simulink model "test_supervisorV2"  (R2023b)
settings: Solver=FixedStepDiscrete  StartTime=0.0  StopTime=inf  FixedStep=1e-3  RelTol=1e-3  EnableMultiTasking=on
undefined symbols (not defined in the file): ControlModes, MotionControlInitConf, SupervisorEvents
libraries: simulink x1
settings Model: DataDictionary=common.sldd  Creator=mfussi  LastModifiedBy=mfussi
settings SolverCC: ConcurrentTasks=on  AutoInsertRateTranBlk=on  InsertRTBMode=Never (minimum delay)
settings DataIOCC: SaveOutput=off  SignalLogging=off  DSMLogging=off  StreamToWks=off  SaveTime=off  ReturnWorkspaceOutputs=off
settings OptimizationCC: DefaultParameterBehavior=Inlined  UseDivisionForNetSlopeComputation=on  GainParamInheritBuiltInType=on  UseFloatMulNetSlope=on  InlineInvariantSignals=on  EnhancedBackFolding=on  NoFixptDivByZeroProtection=on  EfficientFloat2IntCast=on  OptimizeBlockOrder=speed  DifferentSizesBufferReuse=on  OptimizationCustomize=off  EfficientTunableParamExpr=on
settings DebuggingCC: ParameterTunabilityLossMsg=error
settings HardwareCC: ProdBitPerPointer=32  ProdBitPerSizeT=32  ProdBitPerPtrDiffT=32  ProdLargestAtomicInteger=Long  ProdLargestAtomicFloat=Double  ProdWordSize=32  ProdLongLongMode=on  ProdHWDeviceType=ARM Compatible->ARM Cortex-M
settings SFSimCC: MATLABDynamicMemAlloc=off
settings SFSimCC: SimCustomHeaderCode=|
  | #include "rtw_enable_disable_motors.h"
  | #include "rtw_motor_config.h"
settings SFSimCC: SimUserSources=|
  | rtw_enable_disable_motors.c
  | rtw_motor_config.c
settings RTWCC: Description=Embedded Coder  SystemTargetFile=ert.tlc  GenCodeOnly=on  TemplateMakefile=ert_default_tmf  RTWUseSimCustomCode=on
settings RTWCC: CustomHeaderCode=|
  | #include "rtw_enable_disable_motors.h"
  | #include "rtw_motor_config.h"
settings RTWCC: CustomSource=|
  | rtw_enable_disable_motors.c
  | rtw_motor_config.c
settings CodeAppCC: ForceParamTrailComments=on  IgnoreCustomStorageClasses=off  OperatorAnnotations=on  SimulinkDataObjDesc=on  SFDataObjDesc=on  InsertBlockDesc=on
settings ERTTargetCC: TargetLangStandard=C99 (ISO)  CodeReplacementLibrary=ARM Cortex-M,iCubTech  GenerateSampleERTMain=on  SuppressErrorStatus=on  CodeInterfacePackaging=Reusable function  SupportNonFinite=off  InlinedParameterPlacement=NonHierarchical  RootIOFormat=Structure reference  ERTCustomFileTemplate=example_file_process.tlc

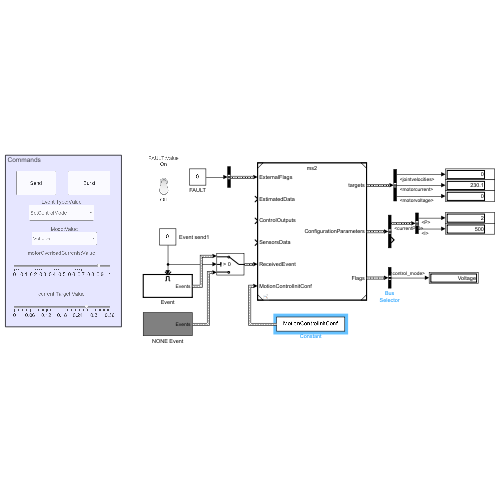
[thumbnail: Simulink's stored preview of the top-level diagram]
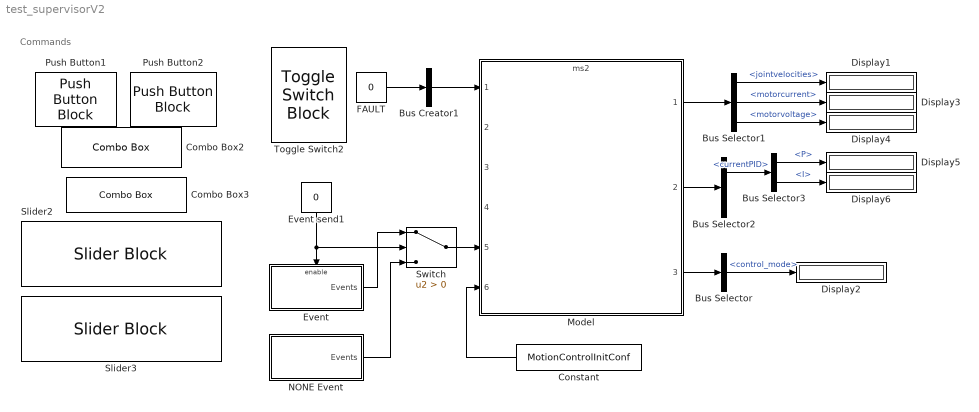
== system test_supervisorV2 ==
  note: Commands
  Bus Creator1 : BusCreator  Inputs=1  OutDataTypeStr=Bus: ExternalFlags  NonVirtualBus=on
      settings: InheritFromInputs=off
  Bus Selector : BusSelector  OutputSignals=control_mode
  Bus Selector1 : BusSelector  OutputSignals=jointvelocities,motorcurrent,motorvoltage
  Bus Selector2 : BusSelector  OutputSignals=pids.currentPID,thresholds
  Bus Selector3 : BusSelector  OutputSignals=P,I
  Combo Box2 : ComboBox  SelectedLabel=SetControlMode  UseEnumeratedDataType=on  EnumeratedDataType=SupervisorEvents
      settings: Values={{'None', 'SetLimit', 'SetControlMode', 'SetMotorConfig', 'SetPid', 'SetTarget'}, [0 1 2 5 3 4]}
  Combo Box3 : ComboBox  SelectedLabel=Voltage  UseEnumeratedDataType=on  EnumeratedDataType=ControlModes
      settings: Values={{'NotConfigured', 'Idle', 'Position', 'PositionDirect', 'Current', 'Velocity', 'Voltage', 'Torque', 'HwFaultCM'}, [0 1 2 3 4 5 6 7 8]}
  Constant : Constant  Value=MotionControlInitConf  OutDataTypeStr=Bus: ActuatorConfiguration
  Display{1..6} (6 alike) : Display
  Event : Subsystem
  Event send1 : Constant  Value=0
  FAULT : Constant  Value=0  OutDataTypeStr=Inherit: Inherit via back propagation
  Model : ModelReference  ModelNameDialog=ms2.slx  SimulationMode=Normal  ModelReferenceVersion=1.148
  NONE Event : Subsystem
  Push Button1 : PushButtonBlock  ButtonText=Send  OffValue=0.000000
  Push Button2 : PushButtonBlock  ButtonText=Burst  ButtonType=Latch  OffValue=0.000000
  Slider2 : SliderBlock  ScaleMax=1
  Slider3 : SliderBlock  ScaleMax=0.36
  Switch : Switch  Criteria=u2 > Threshold  SaturateOnIntegerOverflow=off  InputSameDT=off
  Toggle Switch2 : ToggleSwitchBlock
      settings: Values={{'Off', 'On'}, [0 1]}
  wires:
  Event/1(Events) -> Switch/1
  FAULT/1 -> Bus Creator1/1
  Bus Creator1/1 -> Model/1
  Model/3 -> Bus Selector/1
  Bus Selector/1 -> Display2/1  "<control_mode>"
  Switch/1 -> Model/5
  Event send1/1 -> Switch/2, Event/Enable
  NONE Event/1(Events) -> Switch/3
  Model/1 -> Bus Selector1/1
  Bus Selector1/1 -> Display1/1  "<jointvelocities>"
  Bus Selector1/2 -> Display3/1  "<motorcurrent>"
  Bus Selector1/3 -> Display4/1  "<motorvoltage>"
  Bus Selector2/1 -> Bus Selector3/1  "<currentPID>"
  Constant/1 -> Model/6
  Model/2 -> Bus Selector2/1
  Bus Selector3/1 -> Display5/1  "<P>"
  Bus Selector3/2 -> Display6/1  "<I>"

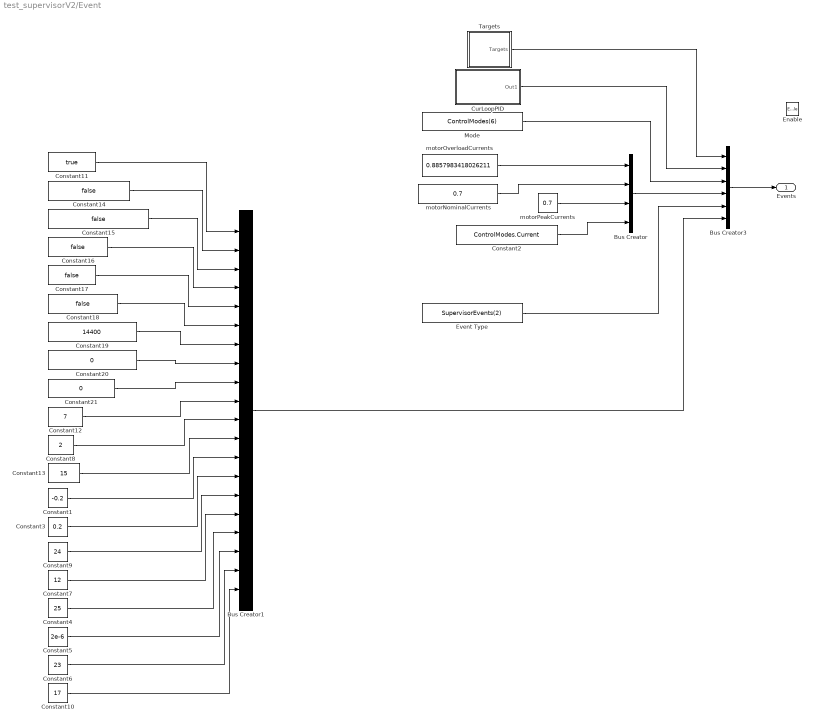
== system test_supervisorV2/Event ==
  Enable : EnablePort
  Bus Creator : BusCreator  Inputs=4  OutDataTypeStr=Bus: SupervisorInputLimits
  Bus Creator1 : BusCreator  Inputs=20  OutDataTypeStr=Bus: MotorConfiguration  NonVirtualBus=on
      settings: InheritFromInputs=off
  Bus Creator3 : BusCreator  Inputs=6  OutDataTypeStr=Bus: SupervisorReceivedEvents  NonVirtualBus=on
      settings: InheritFromInputs=off
  Constant1 : Constant  Value=-0.2  OutDataTypeStr=single
  Constant10 : Constant  Value=17  OutDataTypeStr=single
  Constant11 : Constant  Value=true  OutDataTypeStr=boolean
  Constant12 : Constant  Value=7  OutDataTypeStr=uint8
  Constant13 : Constant  Value=15  OutDataTypeStr=single
  Constant{14..18} (5 alike) : Constant  Value=false  OutDataTypeStr=boolean
  Constant19 : Constant  Value=14400  OutDataTypeStr=int16
  Constant2 : Constant  Value=ControlModes.Current  OutDataTypeStr=Enum: ControlModes
  Constant20 : Constant  Value=0  OutDataTypeStr=int16
  Constant21 : Constant  Value=0  OutDataTypeStr=uint8
  Constant3 : Constant  Value=0.2  OutDataTypeStr=single
  Constant4 : Constant  Value=25  OutDataTypeStr=single
  Constant5 : Constant  Value=2e-6  OutDataTypeStr=single
  Constant6 : Constant  Value=23  OutDataTypeStr=single
  Constant7 : Constant  Value=12  OutDataTypeStr=single
  Constant8 : Constant  Value=2  OutDataTypeStr=single
  Constant9 : Constant  Value=24  OutDataTypeStr=single
  CurLoopPID : Subsystem  mask{OutMax=0, OutMin=0, P=2, I=500, D=0, N=10, I0=0, D0=0, shift_factor=0}
      mask prompts: shift_factor "Shift Factor"
  Event Type : Constant  Value=SupervisorEvents(2)  OutDataTypeStr=Enum: SupervisorEvents
  Mode : Constant  Value=ControlModes(6)  OutDataTypeStr=Enum: ControlModes
  Targets : Subsystem
  motorNominalCurrents : Constant  Value=0.7  OutDataTypeStr=single
  motorOverloadCurrents : Constant  Value=0.8857983418026211  OutDataTypeStr=single
  motorPeakCurrents : Constant  Value=0.7  OutDataTypeStr=single
  Events : Outport  OutDataTypeStr=Bus: SupervisorReceivedEvents
  wires:
  Bus Creator/1 -> Bus Creator3/4
  Bus Creator1/1 -> Bus Creator3/6
  Mode/1 -> Bus Creator3/3
  Targets/1(Targets) -> Bus Creator3/1
  Event Type/1 -> Bus Creator3/5
  CurLoopPID/1(Out1) -> Bus Creator3/2
  motorPeakCurrents/1 -> Bus Creator/3
  Constant2/1 -> Bus Creator/4
  motorOverloadCurrents/1 -> Bus Creator/1
  motorNominalCurrents/1 -> Bus Creator/2
  Bus Creator3/1 -> Events/1
  Constant4/1 -> Bus Creator1/17
  Constant6/1 -> Bus Creator1/19
  Constant17/1 -> Bus Creator1/5
  Constant14/1 -> Bus Creator1/2
  Constant8/1 -> Bus Creator1/11
  Constant10/1 -> Bus Creator1/20
  Constant5/1 -> Bus Creator1/18
  Constant11/1 -> Bus Creator1/1
  Constant1/1 -> Bus Creator1/13
  Constant7/1 -> Bus Creator1/16
  Constant9/1 -> Bus Creator1/15
  Constant3/1 -> Bus Creator1/14
  Constant16/1 -> Bus Creator1/4
  Constant13/1 -> Bus Creator1/12
  Constant18/1 -> Bus Creator1/6
  Constant21/1 -> Bus Creator1/9
  Constant12/1 -> Bus Creator1/10
  Constant19/1 -> Bus Creator1/7
  Constant20/1 -> Bus Creator1/8
  Constant15/1 -> Bus Creator1/3

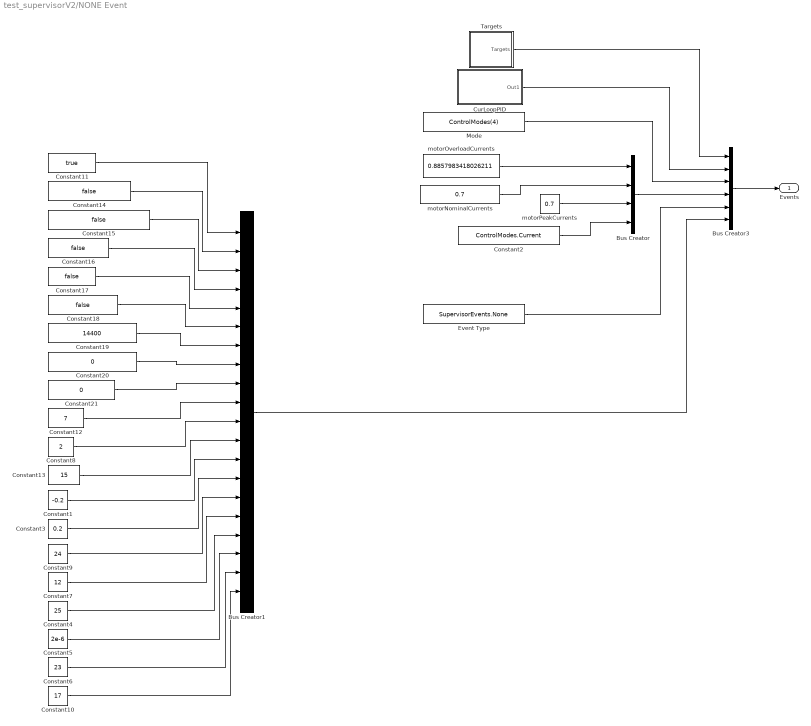
== system test_supervisorV2/NONE Event ==
  Bus Creator : BusCreator  Inputs=4  OutDataTypeStr=Bus: SupervisorInputLimits
  Bus Creator1 : BusCreator  Inputs=20  OutDataTypeStr=Bus: MotorConfiguration  NonVirtualBus=on
      settings: InheritFromInputs=off
  Bus Creator3 : BusCreator  Inputs=6  OutDataTypeStr=Bus: SupervisorReceivedEvents  NonVirtualBus=on
      settings: InheritFromInputs=off
  Constant1 : Constant  Value=-0.2  OutDataTypeStr=single
  Constant10 : Constant  Value=17  OutDataTypeStr=single
  Constant11 : Constant  Value=true  OutDataTypeStr=boolean
  Constant12 : Constant  Value=7  OutDataTypeStr=uint8
  Constant13 : Constant  Value=15  OutDataTypeStr=single
  Constant{14..18} (5 alike) : Constant  Value=false  OutDataTypeStr=boolean
  Constant19 : Constant  Value=14400  OutDataTypeStr=int16
  Constant2 : Constant  Value=ControlModes.Current  OutDataTypeStr=Enum: ControlModes
  Constant20 : Constant  Value=0  OutDataTypeStr=int16
  Constant21 : Constant  Value=0  OutDataTypeStr=uint8
  Constant3 : Constant  Value=0.2  OutDataTypeStr=single
  Constant4 : Constant  Value=25  OutDataTypeStr=single
  Constant5 : Constant  Value=2e-6  OutDataTypeStr=single
  Constant6 : Constant  Value=23  OutDataTypeStr=single
  Constant7 : Constant  Value=12  OutDataTypeStr=single
  Constant8 : Constant  Value=2  OutDataTypeStr=single
  Constant9 : Constant  Value=24  OutDataTypeStr=single
  CurLoopPID : Subsystem  mask{OutMax=0, OutMin=0, P=2, I=500, D=0, N=10, I0=0, D0=0, shift_factor=0}
      mask prompts: shift_factor "Shift Factor"
  Event Type : Constant  Value=SupervisorEvents.None  OutDataTypeStr=Enum: SupervisorEvents
  Mode : Constant  Value=ControlModes(4)  OutDataTypeStr=Enum: ControlModes
  Targets : Subsystem
  motorNominalCurrents : Constant  Value=0.7  OutDataTypeStr=single
  motorOverloadCurrents : Constant  Value=0.8857983418026211  OutDataTypeStr=single
  motorPeakCurrents : Constant  Value=0.7  OutDataTypeStr=single
  Events : Outport  OutDataTypeStr=Bus: SupervisorReceivedEvents
  wires:
  Bus Creator/1 -> Bus Creator3/4
  Bus Creator1/1 -> Bus Creator3/6
  Mode/1 -> Bus Creator3/3
  Targets/1(Targets) -> Bus Creator3/1
  Event Type/1 -> Bus Creator3/5
  CurLoopPID/1(Out1) -> Bus Creator3/2
  motorPeakCurrents/1 -> Bus Creator/3
  Constant2/1 -> Bus Creator/4
  motorOverloadCurrents/1 -> Bus Creator/1
  motorNominalCurrents/1 -> Bus Creator/2
  Bus Creator3/1 -> Events/1
  Constant4/1 -> Bus Creator1/17
  Constant6/1 -> Bus Creator1/19
  Constant17/1 -> Bus Creator1/5
  Constant14/1 -> Bus Creator1/2
  Constant8/1 -> Bus Creator1/11
  Constant10/1 -> Bus Creator1/20
  Constant5/1 -> Bus Creator1/18
  Constant11/1 -> Bus Creator1/1
  Constant1/1 -> Bus Creator1/13
  Constant7/1 -> Bus Creator1/16
  Constant9/1 -> Bus Creator1/15
  Constant3/1 -> Bus Creator1/14
  Constant16/1 -> Bus Creator1/4
  Constant13/1 -> Bus Creator1/12
  Constant18/1 -> Bus Creator1/6
  Constant21/1 -> Bus Creator1/9
  Constant12/1 -> Bus Creator1/10
  Constant19/1 -> Bus Creator1/7
  Constant20/1 -> Bus Creator1/8
  Constant15/1 -> Bus Creator1/3

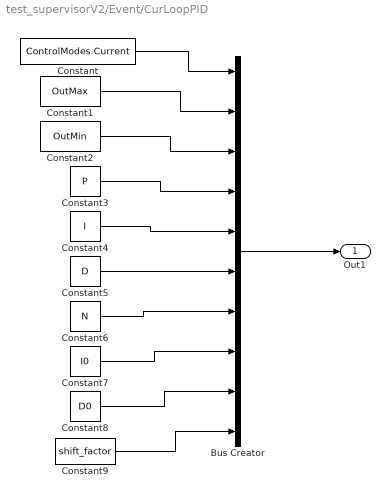
== system test_supervisorV2/Event/CurLoopPID ==
  Bus Creator : BusCreator  Inputs=10  OutDataTypeStr=Bus: PID  NonVirtualBus=on
      settings: InheritFromInputs=off
  Constant : Constant  Value=ControlModes.Current
  Constant1 : Constant  Value=OutMax  OutDataTypeStr=single
  Constant2 : Constant  Value=OutMin  OutDataTypeStr=single
  Constant3 : Constant  Value=P  OutDataTypeStr=single
  Constant4 : Constant  Value=I  OutDataTypeStr=single
  Constant5 : Constant  Value=D  OutDataTypeStr=single
  Constant6 : Constant  Value=N  OutDataTypeStr=single
  Constant7 : Constant  Value=I0  OutDataTypeStr=single
  Constant8 : Constant  Value=D0  OutDataTypeStr=single
  Constant9 : Constant  Value=shift_factor  OutDataTypeStr=uint8
  Out1 : Outport  OutDataTypeStr=Bus: PID
  wires:
  Bus Creator/1 -> Out1/1
  Constant8/1 -> Bus Creator/9
  Constant3/1 -> Bus Creator/4
  Constant5/1 -> Bus Creator/6
  Constant1/1 -> Bus Creator/2
  Constant7/1 -> Bus Creator/8
  Constant2/1 -> Bus Creator/3
  Constant9/1 -> Bus Creator/10
  Constant4/1 -> Bus Creator/5
  Constant/1 -> Bus Creator/1
  Constant6/1 -> Bus Creator/7

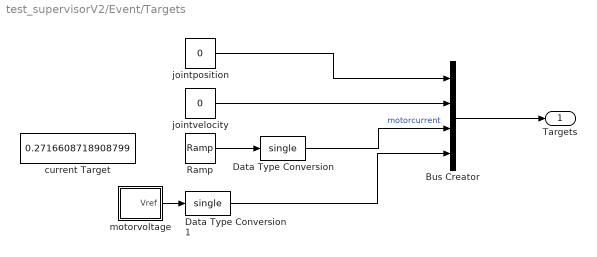
== system test_supervisorV2/Event/Targets ==
  Bus Creator : BusCreator  Inputs=4  OutDataTypeStr=Bus: Targets  NonVirtualBus=on
      settings: InheritFromInputs=off
  Data Type Conversion : DataTypeConversion  OutDataTypeStr=single  SaturateOnIntegerOverflow=off  RndMeth=Floor
  Data Type Conversion1 : DataTypeConversion  OutDataTypeStr=single  SaturateOnIntegerOverflow=off  RndMeth=Floor
  Ramp : simulink/Sources/Ramp  slope=0.1  start=0  InitialOutput=0
  current Target : Constant  Value=0.2716608718908799
  jointposition : Constant  Value=0  OutDataTypeStr=single
  jointvelocity : Constant  Value=0  OutDataTypeStr=single
  motorvoltage : Subsystem
  Targets : Outport
  wires:
  Bus Creator/1 -> Targets/1
  jointposition/1 -> Bus Creator/1
  jointvelocity/1 -> Bus Creator/2
  Data Type Conversion1/1 -> Bus Creator/4
  Data Type Conversion/1 -> Bus Creator/3  "motorcurrent"
  motorvoltage/1(Vref) -> Data Type Conversion1/1
  Ramp/1 -> Data Type Conversion/1

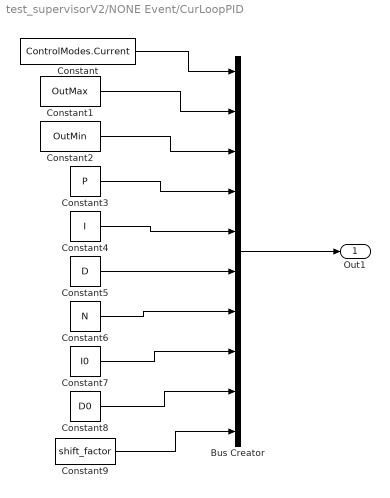
== system test_supervisorV2/NONE Event/CurLoopPID ==
  Bus Creator : BusCreator  Inputs=10  OutDataTypeStr=Bus: PID  NonVirtualBus=on
      settings: InheritFromInputs=off
  Constant : Constant  Value=ControlModes.Current
  Constant1 : Constant  Value=OutMax  OutDataTypeStr=single
  Constant2 : Constant  Value=OutMin  OutDataTypeStr=single
  Constant3 : Constant  Value=P  OutDataTypeStr=single
  Constant4 : Constant  Value=I  OutDataTypeStr=single
  Constant5 : Constant  Value=D  OutDataTypeStr=single
  Constant6 : Constant  Value=N  OutDataTypeStr=single
  Constant7 : Constant  Value=I0  OutDataTypeStr=single
  Constant8 : Constant  Value=D0  OutDataTypeStr=single
  Constant9 : Constant  Value=shift_factor  OutDataTypeStr=uint8
  Out1 : Outport  OutDataTypeStr=Bus: PID
  wires:
  Bus Creator/1 -> Out1/1
  Constant8/1 -> Bus Creator/9
  Constant3/1 -> Bus Creator/4
  Constant5/1 -> Bus Creator/6
  Constant1/1 -> Bus Creator/2
  Constant7/1 -> Bus Creator/8
  Constant2/1 -> Bus Creator/3
  Constant9/1 -> Bus Creator/10
  Constant4/1 -> Bus Creator/5
  Constant/1 -> Bus Creator/1
  Constant6/1 -> Bus Creator/7

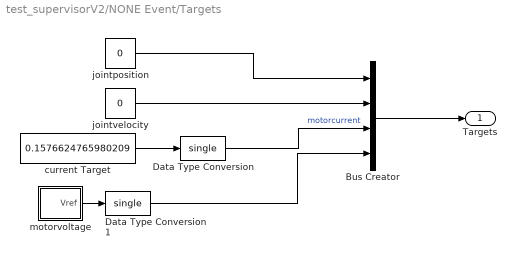
== system test_supervisorV2/NONE Event/Targets ==
  Bus Creator : BusCreator  Inputs=4  OutDataTypeStr=Bus: Targets  NonVirtualBus=on
      settings: InheritFromInputs=off
  Data Type Conversion : DataTypeConversion  OutDataTypeStr=single  SaturateOnIntegerOverflow=off  RndMeth=Floor
  Data Type Conversion1 : DataTypeConversion  OutDataTypeStr=single  SaturateOnIntegerOverflow=off  RndMeth=Floor
  current Target : Constant  Value=0.1576624765980209
  jointposition : Constant  Value=0  OutDataTypeStr=single
  jointvelocity : Constant  Value=0  OutDataTypeStr=single
  motorvoltage : Subsystem
  Targets : Outport
  wires:
  Bus Creator/1 -> Targets/1
  jointposition/1 -> Bus Creator/1
  jointvelocity/1 -> Bus Creator/2
  Data Type Conversion1/1 -> Bus Creator/4
  Data Type Conversion/1 -> Bus Creator/3  "motorcurrent"
  motorvoltage/1(Vref) -> Data Type Conversion1/1
  current Target/1 -> Data Type Conversion/1

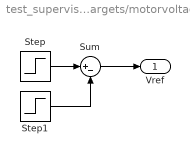
== system test_supervisorV2/Event/Targets/motorvoltage ==
  Step : Step  Time=0.1  After=100
  Step1 : Step  Time=0.2  After=60
  Sum : Sum  Inputs=|+-
  Vref : Outport
  wires:
  Sum/1 -> Vref/1
  Step1/1 -> Sum/2
  Step/1 -> Sum/1

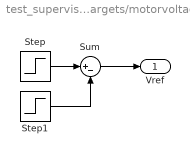
== system test_supervisorV2/NONE Event/Targets/motorvoltage ==
  Step : Step  Time=0.1  After=100
  Step1 : Step  Time=0.2  After=60
  Sum : Sum  Inputs=|+-
  Vref : Outport
  wires:
  Sum/1 -> Vref/1
  Step1/1 -> Sum/2
  Step/1 -> Sum/1
